simulink model "Satellite_Attitude_Control"  (R2022b)
settings: Solver=VariableStepAuto  StartTime=0.0  StopTime=100  RelTol=1e-3
libraries: simulink x3, slpidlib x1
settings Model: Creator=gobis  LastModifiedBy=gobis

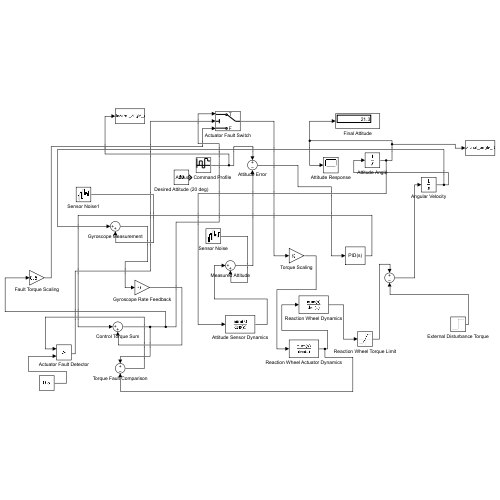
[thumbnail: Simulink's stored preview of the top-level diagram]
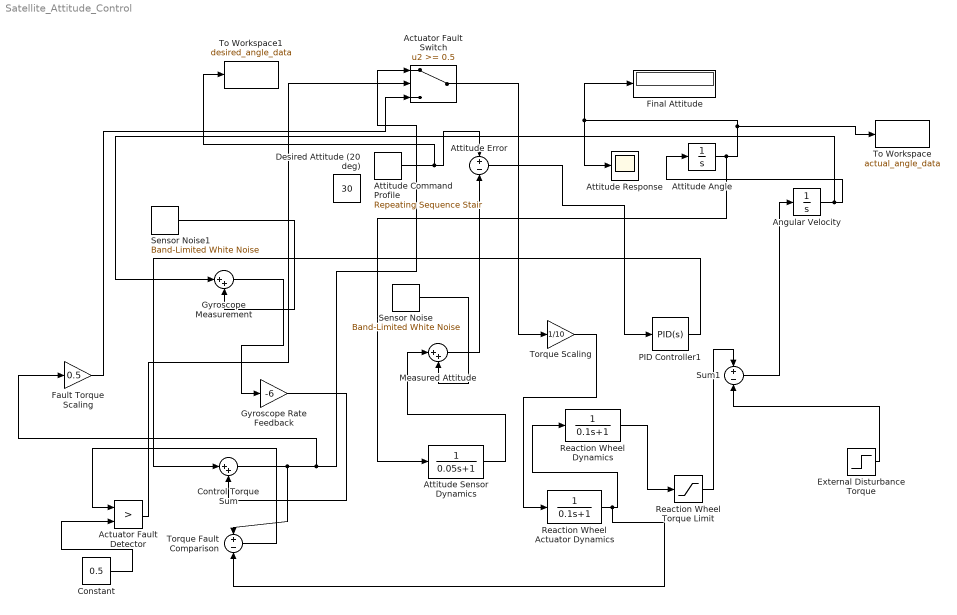
== system Satellite_Attitude_Control ==
  Actuator Fault Detector : RelationalOperator  Operator=>  OutDataTypeStr=boolean  RndMeth=Simplest  InputSameDT=off
  Actuator Fault Switch : Switch  Threshold=0.5  SaturateOnIntegerOverflow=off  InputSameDT=off
  Angular Velocity : Integrator
  Attitude Angle : Integrator
  Attitude Command Profile : simulink/Sources/Repeating Sequence Stair  OutValues=[0 20 -10 30 20]  tsamp=20  OutMin=[]  OutMax=[]  OutDataTypeStr=double  OutputDataTypeScalingMode=double  OutDataType=fixdt(0,8)  ConRadixGroup=Best Precision: Vector-wise  OutScaling=2^-12
  Attitude Error : Sum  Inputs=+-
  Attitude Response : Scope
  Attitude Sensor Dynamics : TransferFcn  Denominator=[0.05 1]
  Constant : Constant  Value=0.5
  Control Torque Sum : Sum  Inputs=|++
  Desired Attitude (20 deg) : Constant  Value=30
  External Disturbance Torque : Step  Time=50  After=5  SampleTime=0
  Fault Torque Scaling : Gain  Gain=0.5
  Final Attitude : Display
  Gyroscope Measurement : Sum  Inputs=|++
  Gyroscope Rate Feedback : Gain  Gain=-6
  Measured Attitude : Sum  Inputs=|++
  PID Controller1 : slpidlib/PID Controller  Controller=PID  Form=Parallel  TimeDomain=Continuous-time  UseExternalTs=off  SampleTime=-1  IntegratorMethod=Forward Euler  FilterMethod=Forward Euler  ControllerParametersSource=internal  P=10  I=0.5  UseKiTs=off  D=0  N=100  UseFilter=on  TunerSelectOption=Transfer Function Based (PID Tuner App)  InitialConditionSource=internal  InitialConditionForIntegrator=0  InitialConditionForFilter=0  DifferentiatorICPrevScaledInput=0  ExternalReset=none  TrackingMode=off  Kt=1  LimitOutput=off  SatLimitsSource=internal  UpperSaturationLimit=inf  LowerSaturationLimit=-inf  LinearizeAsGain=on  AntiWindupMode=none  Kb=1  LimitIntegrator=off  UpperIntegratorSaturationLimit=inf  LowerIntegratorSaturationLimit=-inf  POutMin=[]  POutMax=[]  IOutMin=[]  IOutMax=[]  DOutMin=[]  DOutMax=[]  NOutMin=[]  NOutMax=[]  SumOutMin=[]  SumOutMax=[]  SaturationOutMin=[]  SaturationOutMax=[]  PParamMin=[]  PParamMax=[]  IParamMin=[]  IParamMax=[]  DParamMin=[]  DParamMax=[]  NParamMin=[]  NParamMax=[]  KbParamMin=[]  KbParamMax=[]  KtParamMin=[]  KtParamMax=[]  KbOutMin=[]  KbOutMax=[]  KtOutMin=[]  KtOutMax=[]  IntegratorOutMin=[]  IntegratorOutMax=[]  FilterOutMin=[]  FilterOutMax=[]  SumI1OutMin=[]  SumI1OutMax=[]  SumI2OutMin=[]  SumI2OutMax=[]  SumI3OutMin=[]  SumI3OutMax=[]  SumI4OutMin=[]  SumI4OutMax=[]  SumDOutMin=[]  SumDOutMax=[]  DifferentiatorOutMin=[]  DifferentiatorOutMax=[]  FilterDiffOutCoefMin=[]  FilterDiffOutCoefMax=[]  ReciprocalOutMin=[]  ReciprocalOutMax=[]  SumDenOutMin=[]  SumDenOutMax=[]  SumNumOutMin=[]  SumNumOutMax=[]  DivideOutMin=[]  DivideOutMax=[]  UdiffTsProdOutMin=[]  UdiffTsProdOutMax=[]  NTsProdOutMin=[]  NTsProdOutMax=[]  UintegralTsProdOutMin=[]  UintegralTsProdOutMax=[]  UngainTsProdOutMin=[]  UngainTsProdOutMax=[]  ClampingZeroOutDataTypeStr=Inherit: Inherit via back propagation  ClampingZeroOutMin=[]  ClampingZeroOutMax=[]  FilterDenConstantOutDataTypeStr=Inherit: Inherit via back propagation  FilterDenConstantOutMin=[]  FilterDenConstantOutMax=[]  PCopyOutDataTypeStr=Inherit: Inherit via back propagation  PCopyOutMin=[]  PCopyOutMax=[]  NCopyOutDataTypeStr=Inherit: Inherit via back propagation  NCopyOutMin=[]  NCopyOutMax=[]  IntegratorContinuousStateAttributes=''  IntegratorStateMustResolveToSignalObject=off  IntegratorRTWStateStorageClass=Auto  FilterContinuousStateAttributes=''  FilterStateMustResolveToSignalObject=off  FilterRTWStateStorageClass=Auto  ParallelPVariant=InternalParameters  IdealPVariant=Disabled  IVariant=InternalParameters  DVariant=InternalParameters  IntegratorVariant=Continuous  SatVariant=Disabled  AWVariant=Passthrough  PCopyVariant=Disabled  TRVariant=Disabled  FdbkBlocksVariant=Forward  IdealPFdbkVariant=Disabled  SatFdbkVariant=Disabled  DerivativeFilterVariant=ContFilter  NVariant=InternalParameters  NCopyVariant=Disabled  FilterICVariant=InternalICsFilter  IntegratorICVariant=InternalICs  ExternalResetVariant=Disabled  TRSumVariant=Passthrough  SumFdbkVariant=Disabled  SumVariant=Sum_PID  TsampFilterVariant=InternalTs  TsampNgainVariant=Passthrough  TsampIntegralVariant=Passthrough  ExternalSaturationOutDataTypeStr=Inherit: Same as second input
  Reaction Wheel Actuator Dynamics : TransferFcn  Denominator=[0.1 1]
  Reaction Wheel Dynamics : TransferFcn  Denominator=[0.1 1]
  Reaction Wheel Torque Limit : Saturate  UpperLimit=10  LowerLimit=-10
  Sensor Noise : simulink/Sources/Band-Limited White Noise  Cov=0.01  Ts=0.01  seed=1
  Sensor Noise1 : simulink/Sources/Band-Limited White Noise  Cov=0.001  Ts=0.01  seed=2
  Sum1 : Sum  Inputs=+-
  To Workspace : ToWorkspace  VariableName=actual_angle_data  SaveFormat=Timeseries  SampleTime=-1
  To Workspace1 : ToWorkspace  VariableName=desired_angle_data  SaveFormat=Timeseries  SampleTime=-1
  Torque Fault Comparison : Sum  Inputs=+-
  Torque Scaling : Gain  Gain=1/10
  wires:
  Angular Velocity/1 -> Gyroscope Measurement/1, Attitude Angle/1
  Sum1/1 -> Angular Velocity/1
  Torque Scaling/1 -> Reaction Wheel Actuator Dynamics/1
  Measured Attitude/1 -> Attitude Error/2
  Attitude Error/1 -> PID Controller1/1
  Sensor Noise/1 -> Measured Attitude/2
  Attitude Angle/1 -> Attitude Sensor Dynamics/1, To Workspace/1, Attitude Response/1, Final Attitude/1
  Reaction Wheel Dynamics/1 -> Reaction Wheel Torque Limit/1
  Reaction Wheel Torque Limit/1 -> Sum1/1
  External Disturbance Torque/1 -> Sum1/2
  Attitude Sensor Dynamics/1 -> Measured Attitude/1
  Sensor Noise1/1 -> Gyroscope Measurement/2
  Gyroscope Rate Feedback/1 -> Control Torque Sum/2
  Gyroscope Measurement/1 -> Gyroscope Rate Feedback/1
  Control Torque Sum/1 -> Torque Fault Comparison/1, Fault Torque Scaling/1, Actuator Fault Switch/1
  Actuator Fault Switch/1 -> Torque Scaling/1
  Fault Torque Scaling/1 -> Actuator Fault Switch/3
  PID Controller1/1 -> Control Torque Sum/1
  Reaction Wheel Actuator Dynamics/1 -> Torque Fault Comparison/2, Reaction Wheel Dynamics/1
  Torque Fault Comparison/1 -> Actuator Fault Detector/1
  Constant/1 -> Actuator Fault Detector/2
  Actuator Fault Detector/1 -> Actuator Fault Switch/2
  Attitude Command Profile/1 -> To Workspace1/1, Attitude Error/1
